simulink model "LOISAGA_GARCIA_No2_BlockDiagramAlgebra_Simulink"  (R2023b)
settings: Solver=VariableStepAuto  StartTime=0.0  StopTime=20  RelTol=1e-3
values from neighbouring files (symbols this model uses):
  G1_den = [1 0 0]    [BAES_RAGUSANTE_Block_Diagram_Algebra_NUMBER1_ORIGINAL.m]    (also in BAES_RAGUSANTE_Block_Diagram_Algebra_NUMBER1_REDUCED.m; LOISAGA_GARCIA_BlockDiagramAlgebra_Problem2.m)
  G1_num = [0 1]    [BAES_RAGUSANTE_Block_Diagram_Algebra_NUMBER1_ORIGINAL.m]    (also in BAES_RAGUSANTE_Block_Diagram_Algebra_NUMBER1_REDUCED.m; LOISAGA_GARCIA_BlockDiagramAlgebra_Problem2.m = 1)
  G2_den = [1 1]    [BAES_RAGUSANTE_Block_Diagram_Algebra_NUMBER1_ORIGINAL.m]    (also in BAES_RAGUSANTE_Block_Diagram_Algebra_NUMBER1_REDUCED.m; LOISAGA_GARCIA_BlockDiagramAlgebra_Problem2.m)
  G2_num = [0 1]    [BAES_RAGUSANTE_Block_Diagram_Algebra_NUMBER1_ORIGINAL.m]    (also in BAES_RAGUSANTE_Block_Diagram_Algebra_NUMBER1_REDUCED.m; LOISAGA_GARCIA_BlockDiagramAlgebra_Problem2.m = 1)
  G3_den = [1 0]    [BAES_RAGUSANTE_Block_Diagram_Algebra_NUMBER1_ORIGINAL.m]    (also in BAES_RAGUSANTE_Block_Diagram_Algebra_NUMBER1_REDUCED.m; LOISAGA_GARCIA_BlockDiagramAlgebra_Problem2.m)
  G3_num = [0 1]    [BAES_RAGUSANTE_Block_Diagram_Algebra_NUMBER1_ORIGINAL.m]    (also in BAES_RAGUSANTE_Block_Diagram_Algebra_NUMBER1_REDUCED.m; LOISAGA_GARCIA_BlockDiagramAlgebra_Problem2.m = 1)
  G4_den = [2 0]    [LOISAGA_GARCIA_BlockDiagramAlgebra_Problem2.m]
  G4_num = 1    [LOISAGA_GARCIA_BlockDiagramAlgebra_Problem2.m]
  H1_den = [1 0]    [BAES_RAGUSANTE_Block_Diagram_Algebra_NUMBER1_ORIGINAL.m]    (also in BAES_RAGUSANTE_Block_Diagram_Algebra_NUMBER1_REDUCED.m; LOISAGA_GARCIA_BlockDiagramAlgebra_Problem2.m)
  H1_num = [0 1]    [BAES_RAGUSANTE_Block_Diagram_Algebra_NUMBER1_ORIGINAL.m]    (also in BAES_RAGUSANTE_Block_Diagram_Algebra_NUMBER1_REDUCED.m; LOISAGA_GARCIA_BlockDiagramAlgebra_Problem2.m = 1)
  H2_den = [1 -1]    [BAES_RAGUSANTE_Block_Diagram_Algebra_NUMBER1_ORIGINAL.m]    (also in BAES_RAGUSANTE_Block_Diagram_Algebra_NUMBER1_REDUCED.m; LOISAGA_GARCIA_BlockDiagramAlgebra_Problem2.m)
  H2_num = [0 1]    [BAES_RAGUSANTE_Block_Diagram_Algebra_NUMBER1_ORIGINAL.m]    (also in BAES_RAGUSANTE_Block_Diagram_Algebra_NUMBER1_REDUCED.m; LOISAGA_GARCIA_BlockDiagramAlgebra_Problem2.m = 1)
  H3_den = [1 -2]    [BAES_RAGUSANTE_Block_Diagram_Algebra_NUMBER1_ORIGINAL.m]    (also in BAES_RAGUSANTE_Block_Diagram_Algebra_NUMBER1_REDUCED.m; LOISAGA_GARCIA_BlockDiagramAlgebra_Problem2.m)
  H3_num = [0 1]    [BAES_RAGUSANTE_Block_Diagram_Algebra_NUMBER1_ORIGINAL.m]    (also in BAES_RAGUSANTE_Block_Diagram_Algebra_NUMBER1_REDUCED.m; LOISAGA_GARCIA_BlockDiagramAlgebra_Problem2.m = 1)
  TF_6_den = conv(G1G2G3G4_den,TF_6_den_sum)    [LOISAGA_GARCIA_BlockDiagramAlgebra_Problem2.m]
  TF_6_num = conv(TF_5_num,G1G2G3G4H1_den)    [LOISAGA_GARCIA_BlockDiagramAlgebra_Problem2.m]
settings Model: Creator=acer  LastModifiedBy=acer

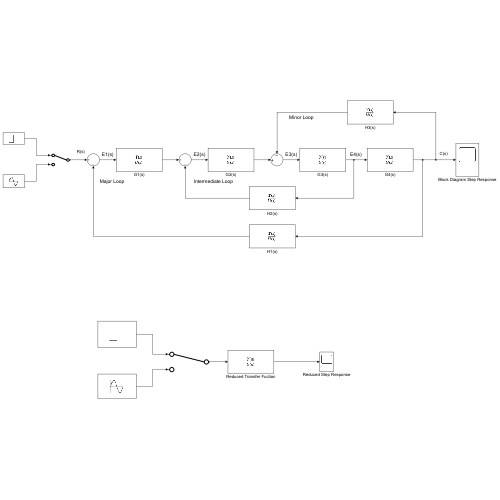
[thumbnail: Simulink's stored preview of the top-level diagram]
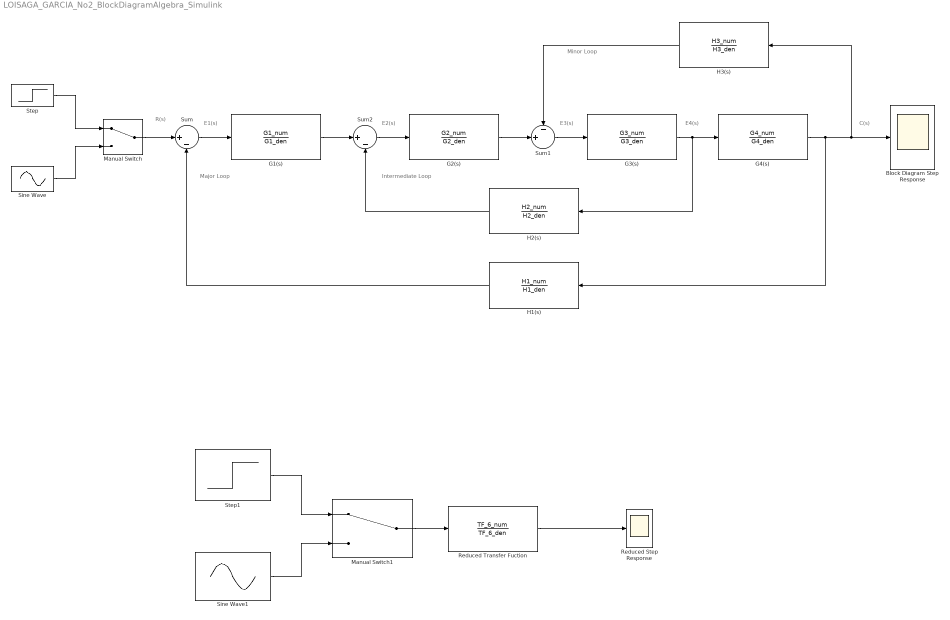
== system LOISAGA_GARCIA_No2_BlockDiagramAlgebra_Simulink ==
  note: E1(s)
  note: Major Loop
  note: Intermediate Loop
  note: Minor Loop
  note: C(s)
  note: R(s)
  note: E2(s)
  note: E3(s)
  note: E4(s)
  Block Diagram Step Response : Scope
  G1(s) : TransferFcn  Numerator=G1_num  Denominator=G1_den
  G2(s) : TransferFcn  Numerator=G2_num  Denominator=G2_den
  G3(s) : TransferFcn  Numerator=G3_num  Denominator=G3_den
  G4(s) : TransferFcn  Numerator=G4_num  Denominator=G4_den
  H1(s) : TransferFcn  Numerator=H1_num  Denominator=H1_den
  H2(s) : TransferFcn  Numerator=H2_num  Denominator=H2_den
  H3(s) : TransferFcn  Numerator=H3_num  Denominator=H3_den
  Manual Switch : ManualSwitch
  Manual Switch1 : ManualSwitch
  Reduced Step Response : Scope
  Reduced Transfer Fuction : TransferFcn  Numerator=TF_6_num  Denominator=TF_6_den
  Sine Wave : Sin  SampleTime=0
  Sine Wave1 : Sin  SampleTime=0
  Step : Step  SampleTime=0
  Step1 : Step  SampleTime=0
  Sum : Sum  Inputs=|+-
  Sum1 : Sum  Inputs=-+|
  Sum2 : Sum  Inputs=|+-
  wires:
  Sum2/1 -> G2(s)/1
  Sum1/1 -> G3(s)/1
  Step/1 -> Manual Switch/1
  Sine Wave/1 -> Manual Switch/2
  Manual Switch/1 -> Sum/1
  Sum/1 -> G1(s)/1
  G2(s)/1 -> Sum1/2
  H3(s)/1 -> Sum1/1
  G1(s)/1 -> Sum2/1
  H2(s)/1 -> Sum2/2
  H1(s)/1 -> Sum/2
  Manual Switch1/1 -> Reduced Transfer Fuction/1
  Reduced Transfer Fuction/1 -> Reduced Step Response/1
  G3(s)/1 -> H2(s)/1, G4(s)/1
  G4(s)/1 -> H1(s)/1, Block Diagram Step Response/1, H3(s)/1
  Sine Wave1/1 -> Manual Switch1/2
  Step1/1 -> Manual Switch1/1
